simulink model "Chen"  (R2014b)
settings: Solver=ode45  StartTime=0.0  StopTime=10.0  RelTol=1e-3
values from neighbouring files (symbols this model uses):
  a = 0.95    [Run_Aizawa.m]    (also in Run_Arneodo.m = -5.5; Run_Chen.m = 33; Run_Chua.m = 15.6; Run_Chua_4D.m = 0.03)
  b = 0.7    [Run_Aizawa.m]    (also in Run_Arneodo.m = 3.5; Run_Chen.m = 3; Run_Chua.m = 28; Run_Duffing.m = 100)
  c = -1    [Run_Arneodo.m]    (also in Run_Chen.m = 25; Run_Chua_4D.m = -1.2; Run_Dadras.m = 2; Run_HindmarshRose.m = 1)
undefined symbols (not defined in the file or in its folder): param
settings Model: Creator=Arek  LastModifiedBy=Arek

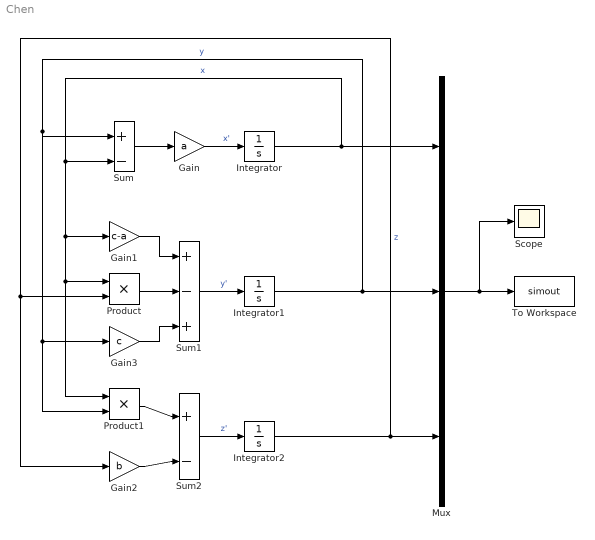
== system Chen ==
  Gain : Gain  Gain=a
  Gain1 : Gain  Gain=c-a
  Gain2 : Gain  Gain=b
  Gain3 : Gain  Gain=c
  Integrator : Integrator  InitialCondition=param.ic(1)
  Integrator1 : Integrator  InitialCondition=param.ic(2)
  Integrator2 : Integrator  InitialCondition=param.ic(3)
  Mux : Mux  Inputs=3
  Product : Product
  Product1 : Product
  Scope : Scope
      settings: ShowLegends=on
  Sum : Sum  Inputs=+|-
  Sum1 : Sum  Inputs=+-+
  Sum2 : Sum  Inputs=+|-
  To Workspace : ToWorkspace  VariableName=simout  SaveFormat=Timeseries  SampleTime=-1
  wires:
  Gain/1 -> Integrator/1  "x'"
  Sum/1 -> Gain/1
  Integrator/1 -> Gain1/1, Product/1, Product1/1, Sum/2, Mux/1  "x"
  Sum1/1 -> Integrator1/1  "y'"
  Integrator1/1 -> Mux/2, Gain3/1, Product1/2, Sum/1  "y"
  Sum2/1 -> Integrator2/1  "z'"
  Product1/1 -> Sum2/1
  Integrator2/1 -> Mux/3, Product/2, Gain2/1  "z"
  Mux/1 -> Scope/1, To Workspace/1
  Gain1/1 -> Sum1/1
  Product/1 -> Sum1/2
  Gain3/1 -> Sum1/3
  Gain2/1 -> Sum2/2
